simulink model "simplified_Z_openloop2015b"  (R2022a)
settings: Solver=VariableStepAuto  StartTime=0.0  StopTime=50  RelTol=1e-3
values from neighbouring files (symbols this model uses):
  mass = 0.2    [simplified_Z_code.m]
  th0 = 0.45    [simplified_Z_code.m]
undefined symbols (not defined in the file or in its folder): DiscIntNeverNeededParam, drone, sigbuilder_block
settings Model: Creator=Jorge Diaz  LastModifiedBy=fades
settings SolverCC: AlgebraicLoopSolver=TrustRegion
settings DataIOCC: ReturnWorkspaceOutputs=off
settings OptimizationCC: LifeSpan=inf
settings DebuggingCC: UnconnectedInputMsg=warning  UnconnectedOutputMsg=warning  UnconnectedLineMsg=warning  SFExecutionAtInitializationDiag=none  SFMachineParentedDataDiag=warning  ArithmeticOperatorsInVariantConditions=warning
settings SFSimCC: SimUseLocalCustomCode=off  CustomCodeUndefinedFunction=UseInterfaceOnly
settings RTWCC: RTWUseLocalCustomCode=off
settings CodeAppCC: StateflowObjectComments=on

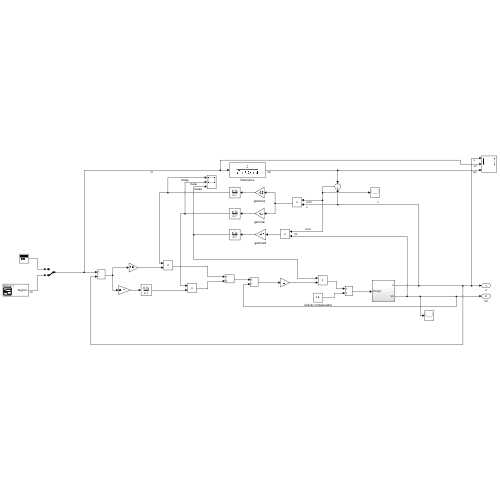
[thumbnail: Simulink's stored preview of the top-level diagram]
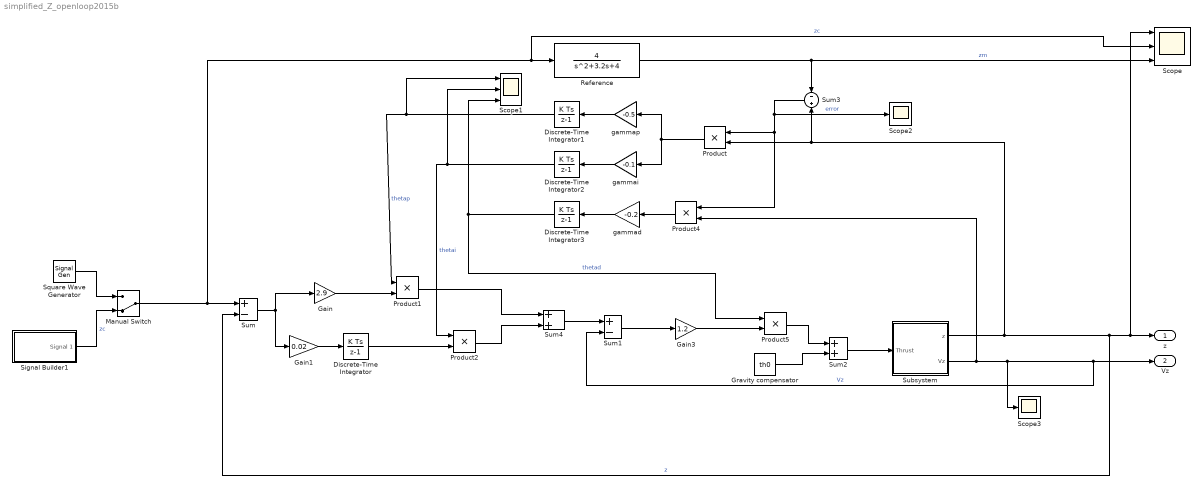
== system simplified_Z_openloop2015b ==
  Discrete-Time Integrator : DiscreteIntegrator  SampleTime=0.02  ICPrevOutput=DiscIntNeverNeededParam  ICPrevScaledInput=DiscIntNeverNeededParam
  Discrete-Time Integrator1 : DiscreteIntegrator  InitialCondition=1  SampleTime=0.02  ICPrevOutput=DiscIntNeverNeededParam  ICPrevScaledInput=DiscIntNeverNeededParam
  Discrete-Time Integrator2 : DiscreteIntegrator  InitialCondition=1  SampleTime=0.02  ICPrevOutput=DiscIntNeverNeededParam  ICPrevScaledInput=DiscIntNeverNeededParam
  Discrete-Time Integrator3 : DiscreteIntegrator  InitialCondition=1  SampleTime=0.02  ICPrevOutput=DiscIntNeverNeededParam  ICPrevScaledInput=DiscIntNeverNeededParam
  Gain : Gain  Gain=2.9
  Gain1 : Gain  Gain=0.02
  Gain3 : Gain  Gain=1.2
  Gravity compensator : Constant  Value=th0
  Manual Switch : ManualSwitch  CurrentSetting=0
  Product{,1..2,4..5} (5 alike) : Product
  Reference : TransferFcn  Numerator=[4]  Denominator=[1 3.2 4]
  Scope : Scope  NumInputPorts=3
  Scope1 : Scope  NumInputPorts=3
  Scope2 : Scope
  Scope3 : Scope
  Signal Builder1 : Subsystem  Tag=STV Subsys  LoadFcn=sigbuilder_block('load');  StartFcn=sigbuilder_block('start');  StopFcn=sigbuilder_block('stop');  ClipboardFcn=sigbuilder_block('clipboard');  mask(Sigbuilder block){tuvar=[0:10]}
      mask help: Simulink:masks:SigbuilderBlock_MD
      mask init:
      | if ~strcmp(get_param(bdroot(gcbh),'SimulationStatus'),'stopped') tuvar = sigbuilder_block('maskInit'); end
      settings: CopyFcn=sigbuilder_block('copy');  DeleteFcn=sigbuilder_block('delete');  ModelCloseFcn=sigbuilder_block('modelClose');  PreSaveFcn=sigbuilder_block('preSave');  PauseFcn=sigbuilder_block('pause');  ContinueFcn=sigbuilder_block('continue');  NameChangeFcn=sigbuilder_block('namechange');  OpenFcn=sigbuilder_block('open',[437.6 199.2 550.4 400 ]);  CloseFcn=sigbuilder_block('close');
      mask Display: plot(0, 0, 100, 100,[2, 2, 32, 32, 2], [68, 8, 8, 68, 68],[32, 2], [38, 38], [32, 19, 2],[53, 60, 44], [32, 17, 17, 2],[16, 16, 31, 31]);txt = getActiveGroup(gcbh);text(2, 100, txt,'verticalAlignment', 'top');
  Square Wave Generator : SignalGenerator  WaveForm=square  Frequency=0.02
  Subsystem : Subsystem
  Sum : Sum  Inputs=+-
  Sum1 : Sum  Inputs=+-
  Sum2 : Sum
  Sum3 : Sum  Inputs=-+
  Sum4 : Sum
  gammad : Gain  Gain=-0.2
  gammai : Gain  Gain=-0.1
  gammap : Gain  Gain=-0.5
  z : Outport
  Vz : Outport  Port=2
  wires:
  Product5/1 -> Sum2/1
  Sum2/1 -> Subsystem/1(Thrust)
  Manual Switch/1 -> Scope/2, Reference/1, Sum/1  "zc"
  Subsystem/1(z) -> Scope/1, z/1, Sum/2, Sum3/2, Product/2  "z"
  Subsystem/2(Vz) -> Product4/2, Scope3/1, Vz/1, Sum1/2  "Vz"
  Sum3/1 -> Product4/1, Product/1, Scope2/1  "error"
  Sum/1 -> Gain1/1, Gain/1
  Reference/1 -> Sum3/1, Scope/3  "zm"
  Gravity compensator/1 -> Sum2/2
  Gain1/1 -> Discrete-Time Integrator/1
  Gain/1 -> Product1/2
  Product2/1 -> Sum4/2
  Product1/1 -> Sum4/1
  Sum4/1 -> Sum1/1
  Product/1 -> gammai/1, gammap/1
  Discrete-Time Integrator/1 -> Product2/2
  Sum1/1 -> Gain3/1
  Gain3/1 -> Product5/2
  gammap/1 -> Discrete-Time Integrator1/1
  Discrete-Time Integrator1/1 -> Scope1/1, Product1/1  "thetap"
  gammai/1 -> Discrete-Time Integrator2/1
  Discrete-Time Integrator2/1 -> Scope1/2, Product2/1  "thetai"
  Product4/1 -> gammad/1
  gammad/1 -> Discrete-Time Integrator3/1
  Discrete-Time Integrator3/1 -> Scope1/3, Product5/1  "thetad"
  Signal Builder1/1(Signal 1) -> Manual Switch/2  "zc"
  Square Wave Generator/1 -> Manual Switch/1

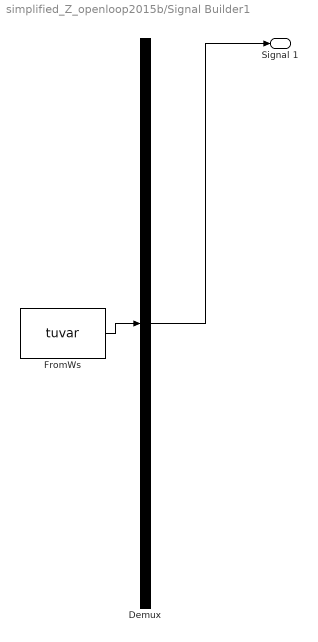
== system simplified_Z_openloop2015b/Signal Builder1 ==
  Demux : Demux  Tag=STV Demux  Outputs=1
      settings: DisplayOption=none
  FromWs : FromWorkspace  Tag=STV FromWs  VariableName=tuvar
      SigBuilderData=|
      | common.afterFinalStr = 'Extrapolate'
      | common.sampleTime = 0
      | dataSet.timeRange = [0 37]
      | dataSet.name = 'Group 1'
      | sbobj.Groups.Name = 'Group 1'
      | sbobj.Groups.Signals.Name = 'Signal 1'
      | sbobj.Groups.Signals.XData = [0 1 1 11 11 21 31 37]
      | sbobj.Groups.Signals.YData = [0 0 1.5 1.5 2 2 0 0]
      | sbobj.Groups.TimeRange = [0 37]
  Signal 1 : Outport  Tag=STV Outport
  wires:
  Demux/1 -> Signal 1/1
  FromWs/1 -> Demux/1

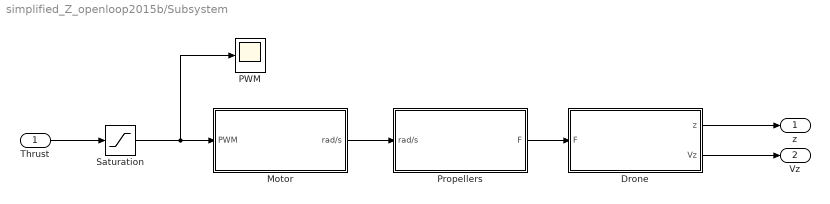
== system simplified_Z_openloop2015b/Subsystem ==
  Thrust : Inport
  Drone : Subsystem
  Motor : Subsystem
  PWM : Scope
  Propellers : Subsystem
  Saturation : Saturate  UpperLimit=0.8  LowerLimit=0.2
  z : Outport
  Vz : Outport  Port=2
  wires:
  Drone/2(Vz) -> Vz/1
  Saturation/1 -> PWM/1, Motor/1(PWM)
  Motor/1(rad/s) -> Propellers/1(rad/s)
  Drone/1(z) -> z/1
  Propellers/1(F) -> Drone/1(F)
  Thrust/1 -> Saturation/1

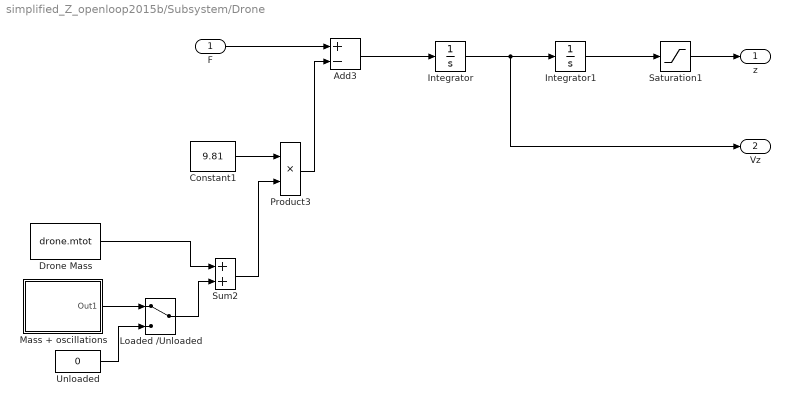
== system simplified_Z_openloop2015b/Subsystem/Drone ==
  F : Inport
  Add3 : Sum  Inputs=+-
  Constant1 : Constant  Value=9.81
  Drone Mass : Constant  Value=drone.mtot
  Integrator : Integrator
  Integrator1 : Integrator
  Loaded /Unloaded : ManualSwitch
  "Mass + oscillations " : Subsystem
  Product3 : Product  Inputs=**
  Saturation1 : Saturate  UpperLimit=inf  LowerLimit=0
  Sum2 : Sum
  Unloaded : Constant  Value=0
  z : Outport
  Vz : Outport  Port=2
  wires:
  Add3/1 -> Integrator/1
  Integrator1/1 -> Saturation1/1
  F/1 -> Add3/1
  Constant1/1 -> Product3/1
  Drone Mass/1 -> Sum2/1
  Sum2/1 -> Product3/2
  Unloaded/1 -> Loaded /Unloaded/2
  Loaded /Unloaded/1 -> Sum2/2
  "Mass + oscillations "/1(Out1) -> Loaded /Unloaded/1
  Product3/1 -> Add3/2
  Saturation1/1 -> z/1
  Integrator/1 -> Vz/1, Integrator1/1

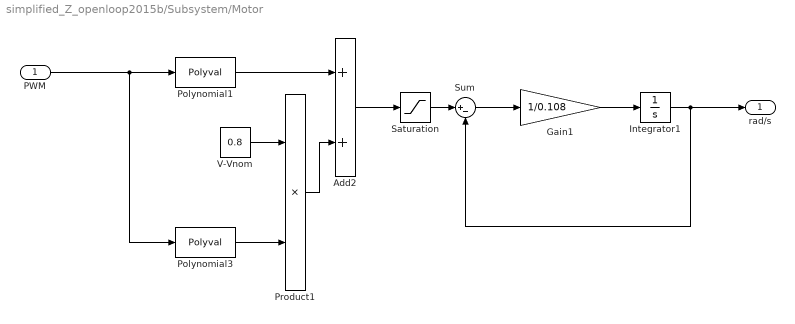
== system simplified_Z_openloop2015b/Subsystem/Motor ==
  PWM : Inport
  Add2 : Sum
  Gain1 : Gain  Gain=1/0.108
  Integrator1 : Integrator
  Polynomial1 : Polyval  Coefs="1.0e+05*[0.5425   -1.9096    2.7131   -1.9927    0.8028   -0.1755    0.0275    0.0000]"
  Polynomial3 : Polyval  Coefs="1.0e+04*[-1.5881    4.7590   -5.6436    3.3845   -1.0784    0.1733   -0.0159    0.0000]"
  Product1 : Product
  Saturation : Saturate  UpperLimit=600  LowerLimit=0
  Sum : Sum  Inputs=|+-
  V-Vnom : Constant  Value=0.8
  rad/s : Outport
  wires:
  PWM/1 -> Polynomial1/1, Polynomial3/1
  Polynomial1/1 -> Add2/1
  Product1/1 -> Add2/2
  V-Vnom/1 -> Product1/1
  Polynomial3/1 -> Product1/2
  Add2/1 -> Saturation/1
  Saturation/1 -> Sum/1
  Sum/1 -> Gain1/1
  Gain1/1 -> Integrator1/1
  Integrator1/1 -> Sum/2, rad/s/1

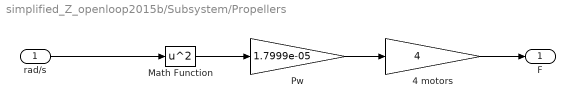
== system simplified_Z_openloop2015b/Subsystem/Propellers ==
  rad/s : Inport
  4 motors : Gain  Gain=4
  Math Function : Math  Operator=square  SignedPower=on
  Pw : Gain  Gain=1.7999e-05
  F : Outport
  wires:
  rad/s/1 -> Math Function/1
  4 motors/1 -> F/1
  Pw/1 -> 4 motors/1
  Math Function/1 -> Pw/1

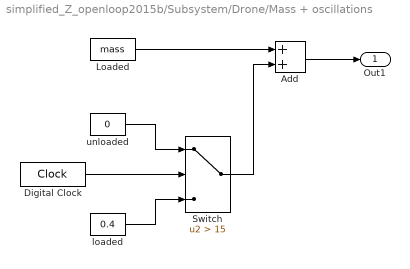
== system simplified_Z_openloop2015b/Subsystem/Drone/Mass + oscillations  ==
  Add : Sum
  Digital Clock : DigitalClock
  Loaded : Constant  Value=mass
  Switch : Switch  Criteria=u2 > Threshold  Threshold=15  SaturateOnIntegerOverflow=off  InputSameDT=off
  "loaded " : Constant  Value=0.4
  unloaded : Constant  Value=0
  Out1 : Outport
  wires:
  Loaded/1 -> Add/1
  Add/1 -> Out1/1
  unloaded/1 -> Switch/1
  Switch/1 -> Add/2
  Digital Clock/1 -> Switch/2
  "loaded "/1 -> Switch/3
